simulink model "sealed_box_example"  (R2023b)
settings: Solver=VariableStepAuto  StartTime=0.0  StopTime=10.0  RelTol=1e-3  AbsTol=1e-3
libraries: acoustical_lib x4, fl_lib x3, nesl_utility x3
settings Model: Creator=steve  LastModifiedBy=steve
settings SolverCC: AutoScaleAbsTol=off  AlgebraicLoopSolver=TrustRegion  MaxZcPerStep=1
settings DebuggingCC: UnconnectedInputMsg=warning  UnconnectedOutputMsg=warning  UnconnectedLineMsg=warning  SymbolicDimsDataTypeCodeGenerationDiagnostic=none
settings ModelReferenceCC: EnableRefExpFcnMdlSchedulingChecks=on
settings SFSimCC: CustomCodeUndefinedFunction=UseInterfaceOnly
settings RTWCC: DLArmComputeVersion=19.05
settings SimscapeCC: SimscapeLogType=all  SimscapeLogSimulationStatistics=on  SimscapeLogDataHistory=10000

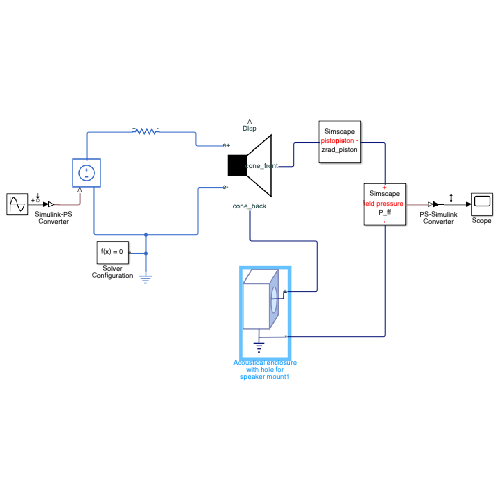
[thumbnail: Simulink's stored preview of the top-level diagram]
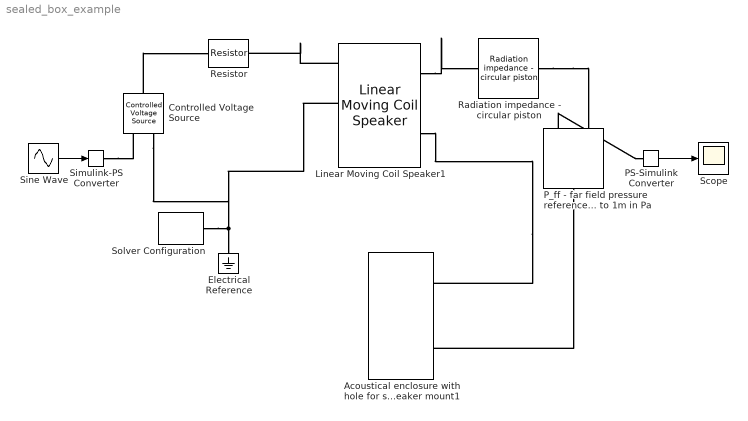
== system sealed_box_example ==
  Acoustical enclosure with hole for speaker mount1 : acoustical_lib/Enclosures/Acoustical enclosure with hole for speaker mount  vol=2.5 l  Sd=30.4 cm^2
      settings: SourceProductName=Acoustical  InternalSimscapePortConfiguration="{\"Bottom\":[],\"Left\":[],\"Right\":[{\"id\":\"pp\",\"label\":\"+\",\"type\":\"acoustical.acoustical\"},{\"id\":\"nn\",\"label\":\"-\",\"type\":\"acoustical.acoustical\"}],\"Top\":[]}"
  Controlled Voltage Source : fl_lib/Electrical/Electrical Sources/Controlled Voltage Source
  Electrical Reference : fl_lib/Electrical/Electrical Elements/Electrical Reference
  Linear Moving Coil Speaker1 : acoustical_lib/Moving Coil Speakers/Linear Moving Coil Speaker  Re=7.8 Ohm  l=1.24*0.1 mH  R2L2=acoustical.enum.R2L2.simple  R2=3.52 Ohm  L2=0.84 mH  mass=4.8 g  Sd=30.4 cm^2  Rm=0.1 N*s/m  BL=5.34 N/A  K=1000 N/m  MechPort=acoustical.enum.WithMechanicalPort.noPort
      settings: SourceProductName=Acoustical  InternalSimscapePortConfiguration="{\"Bottom\":[{\"id\":\"a1\",\"label\":\"cone_back\",\"type\":\"acoustical.acoustical\"}],\"Left\":[{\"id\":\"e0\",\"label\":\"e+\",\"type\":\"foundation.electrical.electrical\"},{\"id\":\"e1\",\"label\":\"e-\",\"type\":\"foundation.electrical.electrical\"}],\"Right\":[{\"id\":\"a0\",\"label\":\"cone_front\",\"type\":\"acoustical.acoustical\"}],\"Top\":[{\"id\":\"Disp\",\"label\":\"Disp\",\"type\":\"output\"}]}"
  PS-Simulink Converter : nesl_utility/PS-Simulink Converter  PhysicalDomain=network_engine_domain  SubClassName=ps_output  LeftPortType=input  RightPortType=output  PseudoPeriodic=off  Frequencies=[]  VectorFormat=inherit  Unit=inherit  AffineConversion=off
  P_ff - far field pressure referenced to 1m in Pa : acoustical_lib/Acoustical Elements/P_ff - far field pressure referenced to 1m in Pa  dist=1 m  u_specify=off  u_priority=None  u=0 m^3/s  u_nominal_specify=off  u_nominal_unit=m^3/s  u_nominal_value=1  p_specify=off  p_priority=None  p=0 Pa  p_nominal_specify=off  p_nominal_unit=Pa  p_nominal_value=1
      settings: SourceProductName=Acoustical  InternalSimscapePortConfiguration="{\"Bottom\":[],\"Left\":[{\"id\":\"pp\",\"label\":\"+\",\"type\":\"acoustical.acoustical\"}],\"Right\":[{\"id\":\"nn\",\"label\":\"-\",\"type\":\"acoustical.acoustical\"}],\"Top\":[{\"id\":\"p_ff\",\"label\":\"far field pressure\",\"type\":\"output\"}]}"
  Radiation impedance - circular piston : acoustical_lib/Acoustical Elements/Radiation impedance - circular piston  Sd=30.4 cm^2
      settings: SourceProductName=Acoustical  InternalSimscapePortConfiguration="{\"Bottom\":[],\"Left\":[{\"id\":\"pa\",\"label\":\"piston +\",\"type\":\"acoustical.acoustical\"}],\"Right\":[{\"id\":\"na\",\"label\":\"piston -\",\"type\":\"acoustical.acoustical\"}],\"Top\":[]}"
  Resistor : fl_lib/Electrical/Electrical Elements/Resistor  R=1 Ohm  i_specify=off  i_priority=None  i=0 A  i_nominal_specify=off  i_nominal_unit=A  i_nominal_value=1  v_specify=off  v_priority=None  v=0 V  v_nominal_specify=off  v_nominal_unit=V  v_nominal_value=1
  Scope : Scope
  Simulink-PS Converter : nesl_utility/Simulink-PS Converter  PhysicalDomain=network_engine_domain  SubClassName=ps_input  LeftPortType=input  RightPortType=output  PseudoPeriodic=off  Frequencies=[]  NoiseDistribution=none  NoiseParameters=[]  Unit=1  AffineConversion=off  FilteringAndDerivatives=provide  SimscapeFilterOrder=1  InputFilterTimeConstant=0.001  UdotUserProvided=0
  Sine Wave : Sin  SampleTime=0
  Solver Configuration : nesl_utility/Solver Configuration  PhysicalDomain=network_engine_domain  SubClassName=solver  LeftPortType=input  RightPortType=generic  Tones=[]  Harmonics=[]  SimulateNoise=off  Profile=off  UseLocalSampling=off  EnableSwitchedLinearOptims=on  FrequencyDomain=off  UseCCode=off  RelTol=0.001  AbsTol=1e-06  MinStep=1e-09  ToWorkspace=off  RevertToSquareIcSolve=off  NumHomotopyIterations=100  PhasorMode=off  PhasorModeNumHarmonics=1  ConsistencySolver=NEWTON_XTOL_AFTER_FTOL  IndexReductionMethod=DerivativeReplacement  DoDC=off  ResidualTolerance=1e-09  ConsistencyTolSource=GLOBAL  ConsistencyAbsTol=0.001  ConsistencyRelTol=0.001  ConsistencyTolFactor=0.001  UseLocalSolver=off  LocalSolverChoice=NE_BACKWARD_EULER_ADVANCER  ResolveIndetEquations=on  FunctionEvalNumThread=1  LocalSolverSampleTime=0.001  DoFixedCost=off  MaxNonlinIter=3  MaxModeIter=2  ComputeImpulses=off  ImpulseIterations=2  LinearAlgebra=auto  LinearAlgebraNumThread=0  EquationFormulation=NE_TIME_EF  DelaysMemoryBudget=1024  AutomaticFiltering=on  FilteringTimeConstant=0.001  PartitionStorageMethod=AS_NEEDED  PartitionMemoryBudget=1024  PartitionMethod=ROBUST  MultibodyUseLocalSolver=off  MultibodyLocalSolverChoice=ODE1  MultibodyLocalSolverSampleTime=0.001
  wires:
  PS-Simulink Converter/1 -> Scope/1
  Sine Wave/1 -> Simulink-PS Converter/1
  connections:
  Controlled Voltage Source/LConn1 -- Resistor/LConn1
  Linear Moving Coil Speaker1/LConn1 -- Resistor/RConn1
  Linear Moving Coil Speaker1/LConn2 -- Controlled Voltage Source/RConn2 -- Solver Configuration/RConn1 -- Electrical Reference/LConn1
  Linear Moving Coil Speaker1/RConn2 -- Acoustical enclosure with hole for speaker mount1/RConn1
  Linear Moving Coil Speaker1/RConn1 -- Radiation impedance - circular piston/LConn1
  Radiation impedance - circular piston/RConn1 -- P_ff - far field pressure referenced to 1m in Pa/LConn1
  P_ff - far field pressure referenced to 1m in Pa/RConn1 -- Acoustical enclosure with hole for speaker mount1/RConn2
  Simulink-PS Converter/RConn1 -- Controlled Voltage Source/RConn1
  P_ff - far field pressure referenced to 1m in Pa/LConn2 -- PS-Simulink Converter/LConn1
